simulink model "SimulationGuidedRecoveryV2_with_drag"  (R2024b)
settings: Solver=VariableStepAuto  StartTime=0.0  StopTime=1500  RelTol=1e-3
libraries: slpidlib x1
settings Model: Creator=Jerry Gao  LastModifiedBy=bgbg0
settings RTWCC: GPUComputeCapability=3.5

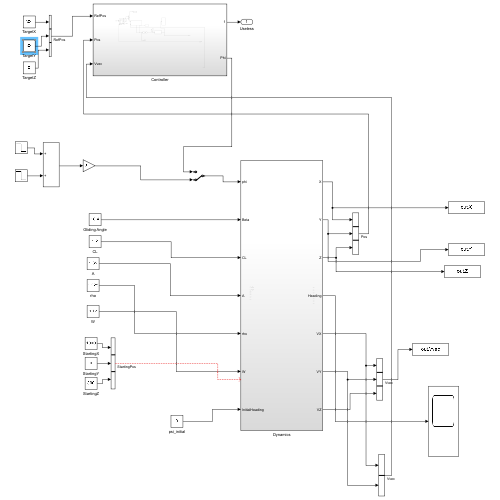
[thumbnail: Simulink's stored preview of the top-level diagram]
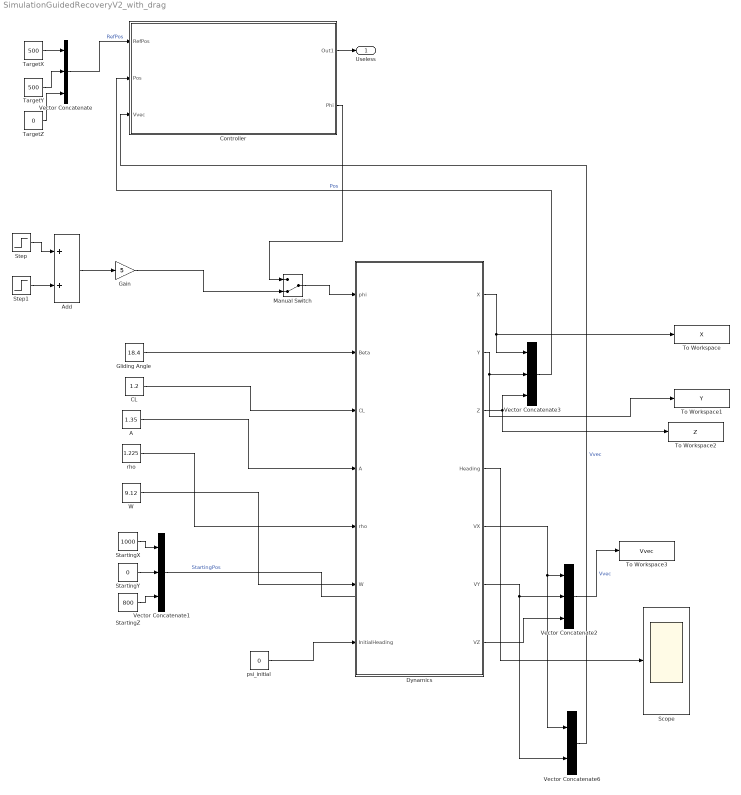
== system SimulationGuidedRecoveryV2_with_drag ==
  A : Constant  Value=1.35
  Add : Sum
  CL : Constant  Value=1.2
  Controller : Subsystem
  Dynamics : Subsystem
  Gain : Gain  Gain=5
  Gliding Angle : Constant  Value=18.4
  Manual Switch : ManualSwitch  CurrentSetting=0
  Scope : Scope
  StartingX : Constant  Value=1000
  StartingY : Constant  Value=0
  StartingZ : Constant  Value=800
  Step : Step  Time=8  Before=1  After=0  SampleTime=0
  Step1 : Step  Time=8  After=-1  SampleTime=0
  TargetX : Constant  Value=500
  TargetY : Constant  Value=500
  TargetZ : Constant  Value=0
  To Workspace : ToWorkspace  VariableName=X  SaveFormat=Timeseries  SampleTime=-1
  To Workspace1 : ToWorkspace  VariableName=Y  SaveFormat=Timeseries  SampleTime=-1
  To Workspace2 : ToWorkspace  VariableName=Z  SaveFormat=Timeseries  SampleTime=-1
  To Workspace3 : ToWorkspace  VariableName=Vvec  SaveFormat=Timeseries  SampleTime=-1
  Vector Concatenate{,1..3} (4 alike) : Concatenate  NumInputs=3
  Vector Concatenate6 : Concatenate
  W : Constant  Value=9.12
  psi_initial : Constant  Value=0
  rho : Constant  Value=1.225
  Useless : Outport
  wires:
  Gliding Angle/1 -> Dynamics/2(Beta)
  CL/1 -> Dynamics/3(CL)
  A/1 -> Dynamics/4(A)
  rho/1 -> Dynamics/5(rho)
  W/1 -> Dynamics/6(W)
  TargetX/1 -> Vector Concatenate/1
  TargetY/1 -> Vector Concatenate/2
  StartingY/1 -> Vector Concatenate1/2
  StartingZ/1 -> Vector Concatenate1/3
  StartingX/1 -> Vector Concatenate1/1
  Vector Concatenate1/1 -> ?  "StartingPos"
  psi_initial/1 -> Dynamics/7(InitialHeading)
  Dynamics/1(X) -> Vector Concatenate3/1, To Workspace/1
  Dynamics/2(Y) -> To Workspace1/1, Vector Concatenate3/2
  Dynamics/4(Heading) -> Scope/1
  Dynamics/3(Z) -> To Workspace2/1, Vector Concatenate3/3
  Dynamics/5(VX) -> Vector Concatenate6/1, Vector Concatenate2/1
  Dynamics/6(VY) -> Vector Concatenate6/2, Vector Concatenate2/2
  Dynamics/7(VZ) -> Vector Concatenate2/3
  Vector Concatenate2/1 -> To Workspace3/1  "Vvec"
  TargetZ/1 -> Vector Concatenate/3
  Vector Concatenate/1 -> Controller/1(RefPos)  "RefPos"
  Vector Concatenate3/1 -> Controller/2(Pos)  "Pos"
  Vector Concatenate6/1 -> Controller/3(Vvec)  "Vvec"
  Controller/1(Out1) -> Useless/1
  Controller/2(Phi) -> Manual Switch/1
  Manual Switch/1 -> Dynamics/1(phi)
  Gain/1 -> Manual Switch/2
  Step/1 -> Add/1
  Step1/1 -> Add/2
  Add/1 -> Gain/1

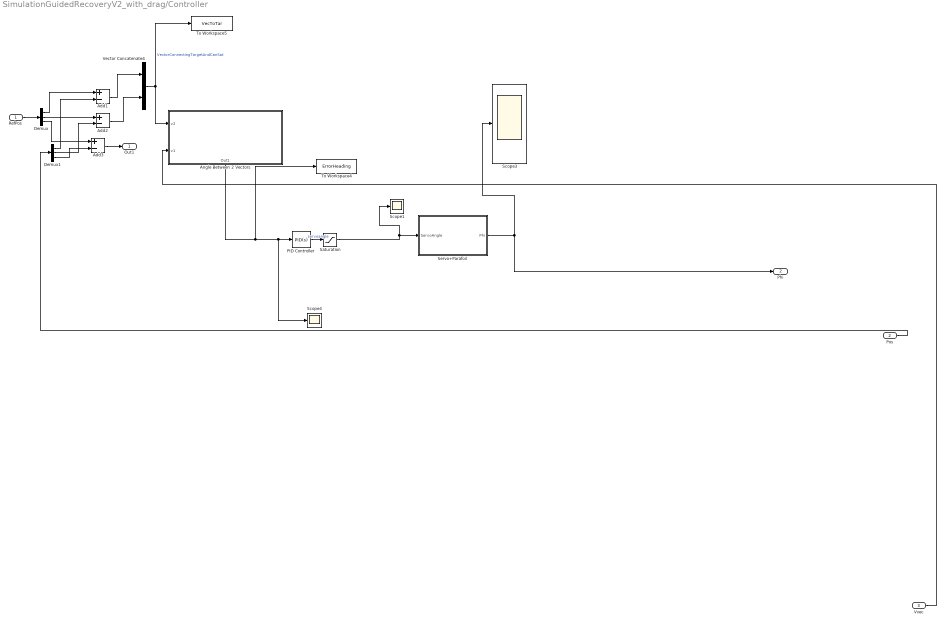
== system SimulationGuidedRecoveryV2_with_drag/Controller ==
  RefPos : Inport
  Pos : Inport  Port=2
  Vvec : Inport  Port=3
  Add1 : Sum  Inputs=+-
  Add2 : Sum  Inputs=+-
  Add3 : Sum  Inputs=+-
  Angle Between 2 Vectors : Subsystem
      settings: PortSchema="{\"entries\":[{\"content\":{\"sides\":[{\"content\":{\"connectorIds\":[\"In1\",\"In2\"]},\"type\":\"ConnectorPlacement.EquallySpacedRectSide\",\"uuid\":\"2a3f35bb-975b-4170-bf2f-b66643bf7732\"},{\"content\":{\"side\":\"RIGHT\"},\"type\":\"ConnectorPlacement.EquallySpacedRectSide\",\"uuid\":\"e83cc06c-abd1-4e89-a0f4-1a246757fc80\"},{\"content\":{\"side\":\"TOP\"},\"type\":\"ConnectorPlacement.EquallySpacedRectSide\",\"uuid\":\"eeba1ec8-f966-4d1c-ad11-91f5f0644dce\"},{\"content\":{\"connectorIds\":[\"Out1\"],\"side\":\"BOTTOM\"},\"type\":\"ConnectorPlacement.EquallySpacedRectSide\",\"uuid\":\"aaaa25ac-3a4f-40f7-9fcb-849203176940\"}]},\"type\":\"ConnectorPlacement.EquallySpacedConnector\",\"uuid\":\"d0b184af-993a-4781-b8c0-335e8ad5db02\"}],\"packageUris\":[\"http://schema.mathworks.com/mf0/Connector/R2020b\"],\"version\":\"1.0\"}"
  Demux : Demux  Outputs=3
  Demux1 : Demux  Outputs=3
  PID Controller : slpidlib/PID Controller  Controller=PID  Form=Parallel  TimeDomain=Continuous-time  UseExternalTs=off  SampleTime=-1  IntegratorMethod=Forward Euler  FilterMethod=Forward Euler  ControllerParametersSource=internal  P=144.769965332485  I=1.05397863888132  UseKiTs=off  D=-31.9542651869893  UseExternalDerivativeSource=off  N=4.53053651790529  UseFilter=on  TunerSelectOption=Transfer Function Based (PID Tuner App)  InitialConditionSource=internal  InitialConditionForIntegrator=0  InitialConditionForFilter=0  DifferentiatorICPrevScaledInput=0  ExternalReset=none  TrackingMode=off  Kt=1  LimitOutput=off  SatLimitsSource=internal  UpperSaturationLimit=inf  LowerSaturationLimit=-inf  LinearizeAsGain=on  AntiWindupMode=none  Kb=1  LimitIntegrator=off  UpperIntegratorSaturationLimit=inf  LowerIntegratorSaturationLimit=-inf  POutMin=[]  POutMax=[]  IOutMin=[]  IOutMax=[]  DOutMin=[]  DOutMax=[]  NOutMin=[]  NOutMax=[]  SumOutMin=[]  SumOutMax=[]  SaturationOutMin=[]  SaturationOutMax=[]  PParamMin=[]  PParamMax=[]  IParamMin=[]  IParamMax=[]  DParamMin=[]  DParamMax=[]  NParamMin=[]  NParamMax=[]  KbParamMin=[]  KbParamMax=[]  KtParamMin=[]  KtParamMax=[]  KbOutMin=[]  KbOutMax=[]  KtOutMin=[]  KtOutMax=[]  IntegratorOutMin=[]  IntegratorOutMax=[]  FilterOutMin=[]  FilterOutMax=[]  SumI1OutMin=[]  SumI1OutMax=[]  SumI2OutMin=[]  SumI2OutMax=[]  SumI3OutMin=[]  SumI3OutMax=[]  SumI4OutMin=[]  SumI4OutMax=[]  SumDOutMin=[]  SumDOutMax=[]  DifferentiatorOutMin=[]  DifferentiatorOutMax=[]  FilterDiffOutCoefMin=[]  FilterDiffOutCoefMax=[]  ReciprocalOutMin=[]  ReciprocalOutMax=[]  SumDenOutMin=[]  SumDenOutMax=[]  SumNumOutMin=[]  SumNumOutMax=[]  DivideOutMin=[]  DivideOutMax=[]  UdiffTsProdOutMin=[]  UdiffTsProdOutMax=[]  NTsProdOutMin=[]  NTsProdOutMax=[]  UintegralTsProdOutMin=[]  UintegralTsProdOutMax=[]  UngainTsProdOutMin=[]  UngainTsProdOutMax=[]  ClampingZeroOutDataTypeStr=Inherit: Inherit via back propagation  ClampingZeroOutMin=[]  ClampingZeroOutMax=[]  FilterDenConstantOutDataTypeStr=Inherit: Inherit via back propagation  FilterDenConstantOutMin=[]  FilterDenConstantOutMax=[]  PCopyOutDataTypeStr=Inherit: Inherit via back propagation  PCopyOutMin=[]  PCopyOutMax=[]  NCopyOutDataTypeStr=Inherit: Inherit via back propagation  NCopyOutMin=[]  NCopyOutMax=[]  IntegratorContinuousStateAttributes=''  IntegratorStateMustResolveToSignalObject=off  IntegratorRTWStateStorageClass=Auto  FilterContinuousStateAttributes=''  FilterStateMustResolveToSignalObject=off  FilterRTWStateStorageClass=Auto  ParallelPVariant=InternalParameters  IdealPVariant=Disabled  IVariant=InternalParameters  DVariant=InternalParameters  IntegratorVariant=Continuous  SatVariant=Disabled  AWVariant=Passthrough  PCopyVariant=Disabled  TRVariant=Disabled  FdbkBlocksVariant=Forward  IdealPFdbkVariant=Disabled  SatFdbkVariant=Disabled  DerivativeFilterVariant=ContFilter  NVariant=InternalParameters  NCopyVariant=Disabled  FilterICVariant=InternalICsFilter  IntegratorICVariant=InternalICs  ExternalResetVariant=Disabled  TRSumVariant=Passthrough  SumFdbkVariant=Disabled  SumVariant=Sum_PID  TsampFilterVariant=InternalTs  TsampNgainVariant=Passthrough  TsampIntegralVariant=Disabled_SignalSpec  ExternalSaturationOutDataTypeStr=Inherit: Same as second input  DerivativeSourceVariant=ErrorSignal  PreIntVariant=InternalPreInt
  Saturation : Saturate  UpperLimit=1260  LowerLimit=-1260
  Scope1 : Scope
  Scope3 : Scope
  Scope4 : Scope
  Servo+Parafoil : Subsystem
  To Workspace4 : ToWorkspace  VariableName=ErrorHeading  SaveFormat=Timeseries  SampleTime=-1
  To Workspace5 : ToWorkspace  VariableName=VecToTar  SaveFormat=Timeseries  SampleTime=-1
  Vector Concatenate4 : Concatenate
  Out1 : Outport
  Phi : Outport  Port=2
  wires:
  Demux/1 -> Add1/1
  Add3/1 -> Out1/1
  PID Controller/1 -> Saturation/1  "servoangle"
  Servo+Parafoil/1(Phi) -> Phi/1, Scope3/1
  RefPos/1 -> Demux/1
  Saturation/1 -> Scope1/1, Servo+Parafoil/1(ServoAngle)
  Vector Concatenate4/1 -> Angle Between 2 Vectors/1(v2), To Workspace5/1  "VectorConnectingTargetAndCanSat"
  Angle Between 2 Vectors/1(Out1) -> PID Controller/1, Scope4/1, To Workspace4/1
  Demux/2 -> Add2/1
  Demux1/2 -> Add2/2
  Demux/3 -> Add3/1
  Add2/1 -> Vector Concatenate4/2
  Add1/1 -> Vector Concatenate4/1
  Demux1/1 -> Add1/2
  Demux1/3 -> Add3/2
  Pos/1 -> Demux1/1
  Vvec/1 -> Angle Between 2 Vectors/2(v1)

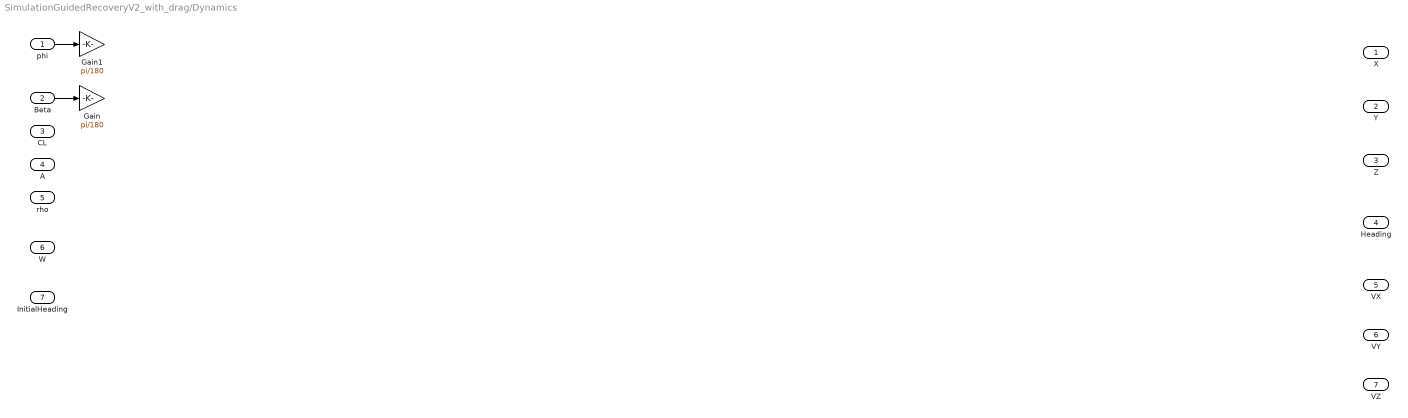
== system SimulationGuidedRecoveryV2_with_drag/Dynamics ==
  phi : Inport
  Beta : Inport  Port=2
  CL : Inport  Port=3
  A : Inport  Port=4
  rho : Inport  Port=5
  W : Inport  Port=6
  InitialHeading : Inport  Port=7
  Gain : Gain  Gain=pi/180
  Gain1 : Gain  Gain=pi/180
  X : Outport
  Y : Outport  Port=2
  Z : Outport  Port=3
  Heading : Outport  Port=4
  VX : Outport  Port=5
  VY : Outport  Port=6
  VZ : Outport  Port=7
  wires:
  Beta/1 -> Gain/1
  phi/1 -> Gain1/1

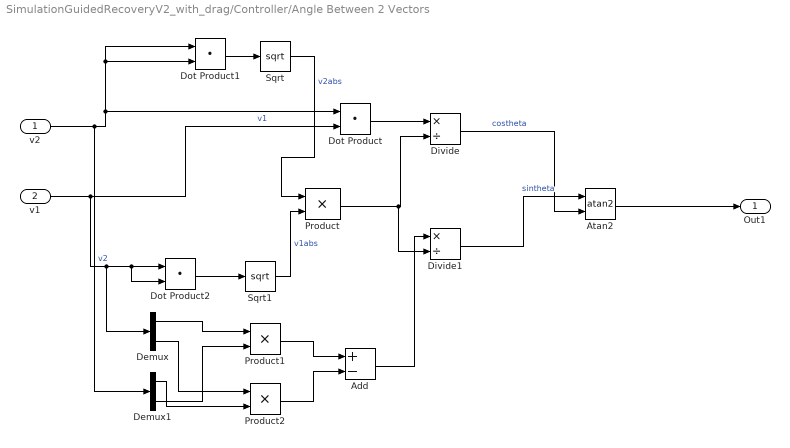
== system SimulationGuidedRecoveryV2_with_drag/Controller/Angle Between 2 Vectors ==
  v2 : Inport
  v1 : Inport  Port=2
  Add : Sum  Inputs=+-
  Atan2 : Trigonometry  Operator=atan2
  Demux : Demux  Outputs=2
  Demux1 : Demux  Outputs=2
  Divide : Product  Inputs=*/
  Divide1 : Product  Inputs=*/
  Dot Product : DotProduct  OutDataTypeStr=Inherit: Inherit via internal rule
  Dot Product1 : DotProduct  OutDataTypeStr=Inherit: Inherit via internal rule
  Dot Product2 : DotProduct  OutDataTypeStr=Inherit: Inherit via internal rule
  Product : Product
  Product1 : Product
  Product2 : Product
  Sqrt : Sqrt
  Sqrt1 : Sqrt
  Out1 : Outport
  wires:
  v1/1 -> Demux/1, Dot Product2/2, Dot Product2/1, Dot Product/2  "v1"
  Dot Product1/1 -> Sqrt/1
  Dot Product2/1 -> Sqrt1/1
  Sqrt/1 -> Product/1  "v2abs"
  Sqrt1/1 -> Product/2  "v1abs"
  Dot Product/1 -> Divide/1
  Product/1 -> Divide1/2, Divide/2
  Divide/1 -> Atan2/2  "costheta"
  v2/1 -> Demux1/1, Dot Product1/2, Dot Product1/1, Dot Product/1  "v2"
  Add/1 -> Divide1/1
  Divide1/1 -> Atan2/1  "sintheta"
  Atan2/1 -> Out1/1
  Demux/1 -> Product1/1
  Demux1/2 -> Product1/2
  Demux/2 -> Product2/1
  Demux1/1 -> Product2/2
  Product1/1 -> Add/1
  Product2/1 -> Add/2

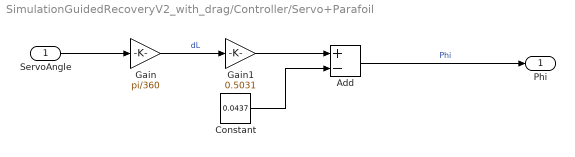
== system SimulationGuidedRecoveryV2_with_drag/Controller/Servo+Parafoil ==
  ServoAngle : Inport
  Add : Sum  Inputs=+-
  Constant : Constant  Value=0.0437
  Gain : Gain  Gain=pi/360
  Gain1 : Gain  Gain=0.5031
  Phi : Outport
  wires:
  ServoAngle/1 -> Gain/1
  Gain/1 -> Gain1/1  "dL"
  Constant/1 -> Add/2
  Gain1/1 -> Add/1
  Add/1 -> Phi/1  "Phi"
